simulink model "simu"  (R2017b)
settings: Solver=ode45  StartTime=0.0  StopTime=20000  MaxStep=1  RelTol=1e-3  AbsTol=1e-6  EnableMultiTasking=on
undefined symbols (not defined in the file): cpp, Cvg, Cvw, dFg, dQg, dTzew, Fg0, K1, Kg, Qg0, rop, t0, Tg0, Twew0, Tzew0
settings Model: Creator=LAB320-1552  LastModifiedBy=kajaczekmackbookpro
settings DataIOCC: LimitDataPoints=on  SaveFormat=Array
settings OptimizationCC: LifeSpan=inf
settings DebuggingCC: UnderspecifiedInitializationDetection=Classic  MergeDetectMultiDrivingBlocksExec=none  StateNameClashWarn=warning  SFUnexpectedBacktrackingDiag=warning  SFNoUnconditionalDefaultTransitionDiag=warning  SFExecutionAtInitializationDiag=none
settings HardwareCC: ProdBitPerPointer=32  ProdBitPerSizeT=32  ProdBitPerPtrDiffT=32  ProdLargestAtomicFloat=None  ProdIntDivRoundTo=Undefined  ProdEndianess=Unspecified  ProdWordSize=32  ProdHWDeviceType=32-bit Generic
settings ModelReferenceCC: PropagateSignalLabelsOutOfModel=off
settings CodeAppCC: StateflowObjectComments=on
settings GRTTargetCC: TargetLangStandard=C89/C90 (ANSI)  GeneratePreprocessorConditionals=Disable all
settings ConfigComp: CovMetricSettings=dw  CovHtmlReporting=on  CovSaveCumulativeToWorkspaceVar=on  CovSaveSingleToWorkspaceVar=on  CovExternalEMLEnable=off

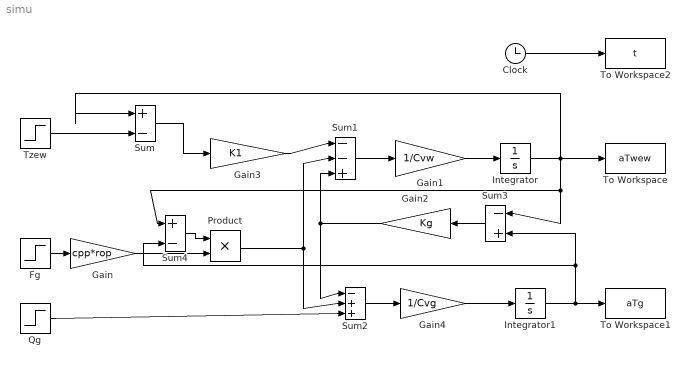
== system simu ==
  Clock : Clock
  Fg : Step  Time=t0  Before=Fg0  After=Fg0+dFg  SampleTime=0
  Gain : Gain  Gain=cpp*rop
  Gain1 : Gain  Gain=1/Cvw
  Gain2 : Gain  Gain=Kg
  Gain3 : Gain  Gain=K1
  Gain4 : Gain  Gain=1/Cvg
  Integrator : Integrator  InitialCondition=Twew0
  Integrator1 : Integrator  InitialCondition=Tg0
  Product : Product
  Qg : Step  Time=t0  Before=Qg0  After=Qg0+dQg  SampleTime=0
  Sum : Sum  Inputs=|+-
  Sum1 : Sum  Inputs=|--+
  Sum2 : Sum  Inputs=|-++
  Sum3 : Sum  Inputs=|-+
  Sum4 : Sum  Inputs=|+-
  To Workspace : ToWorkspace  VariableName=aTwew  SampleTime=-1
  To Workspace1 : ToWorkspace  VariableName=aTg  SampleTime=-1
  To Workspace2 : ToWorkspace  VariableName=t  SampleTime=-1
  Tzew : Step  Time=t0  Before=Tzew0  After=Tzew0+dTzew  SampleTime=0
  wires:
  Gain/1 -> Product/2
  Fg/1 -> Gain/1
  Tzew/1 -> Sum/2
  Gain2/1 -> Sum2/1, Sum1/3
  Product/1 -> Sum1/2, Sum2/2
  Gain3/1 -> Sum1/1
  Sum1/1 -> Gain1/1
  Sum2/1 -> Gain4/1
  Gain4/1 -> Integrator1/1
  Sum3/1 -> Gain2/1
  Gain1/1 -> Integrator/1
  Integrator1/1 -> Sum3/2, Sum4/2, To Workspace1/1
  Clock/1 -> To Workspace2/1
  Qg/1 -> Sum2/3
  Integrator/1 -> Sum/1, Sum3/1, Sum4/1, To Workspace/1
  Sum4/1 -> Product/1
  Sum/1 -> Gain3/1
